simulink model "a2_WH_Help"  (R2018a)
settings: Solver=VariableStepAuto  StartTime=0.0  StopTime=10.0  RelTol=1e-3
settings Model: Creator=burmesdani  LastModifiedBy=burmesdani

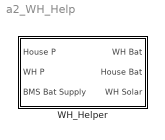
== system a2_WH_Help ==
  WH_Helper : Subsystem

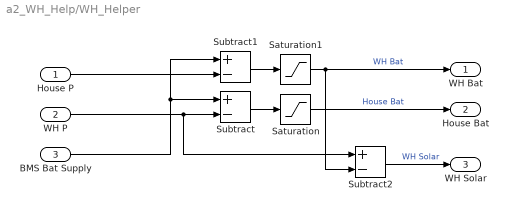
== system a2_WH_Help/WH_Helper ==
  House P : Inport
  WH P : Inport  Port=2
  "BMS Bat Supply " : Inport  Port=3
  Saturation : Saturate  UpperLimit=inf  LowerLimit=0
  Saturation1 : Saturate  UpperLimit=inf  LowerLimit=0
  Subtract : Sum  Inputs=+-
  Subtract1 : Sum  Inputs=+-
  Subtract2 : Sum  Inputs=+-
  WH Bat : Outport
  House Bat : Outport  Port=2
  WH Solar : Outport  Port=3
  wires:
  Subtract2/1 -> WH Solar/1  "WH Solar"
  "BMS Bat Supply "/1 -> Subtract1/1, Subtract/1
  Subtract1/1 -> Saturation1/1
  WH P/1 -> Subtract/2, Subtract2/1
  Subtract/1 -> Saturation/1
  Saturation/1 -> House Bat/1  "House Bat"
  Saturation1/1 -> Subtract2/2, WH Bat/1  "WH Bat"
  House P/1 -> Subtract1/2
